simulink model "ReactionWheel"  (R2024a)
settings: Solver=FixedStepAuto  StartTime=0.0  StopTime=60*60  FixedStep=1  RelTol=1e-3
model workspace (MAT data in the model file):
  I_s = [344.15  0  0; 0  344.15  0; 0  0  688.24]
  LocalBodyOffset = [45 0 0]
undefined symbols (not defined in the file): IAU, juliandate, WMM2020
libraries: aerolibutil x16, sharedtransform x6, aerolibtransform2 x4, matrix_library x4, aerolibconvert2 x4, aerolibatmos2 x1, simulink_extras x1, aerolibsatdyn x1, aerolibobsolete x1, aerolibattitudesys x1, simulink x1, vrlib x1
settings Model: Creator=pierc  LastModifiedBy=pierc

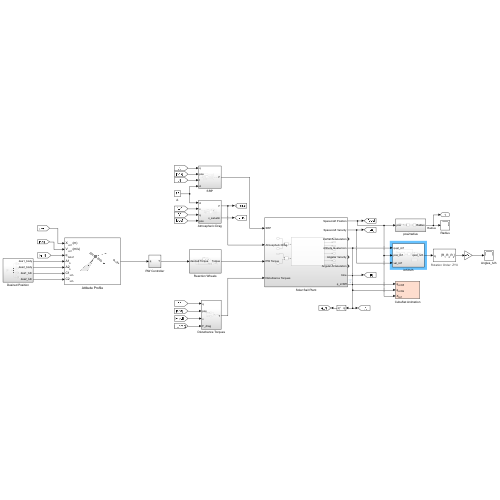
[thumbnail: Simulink's stored preview of the top-level diagram]
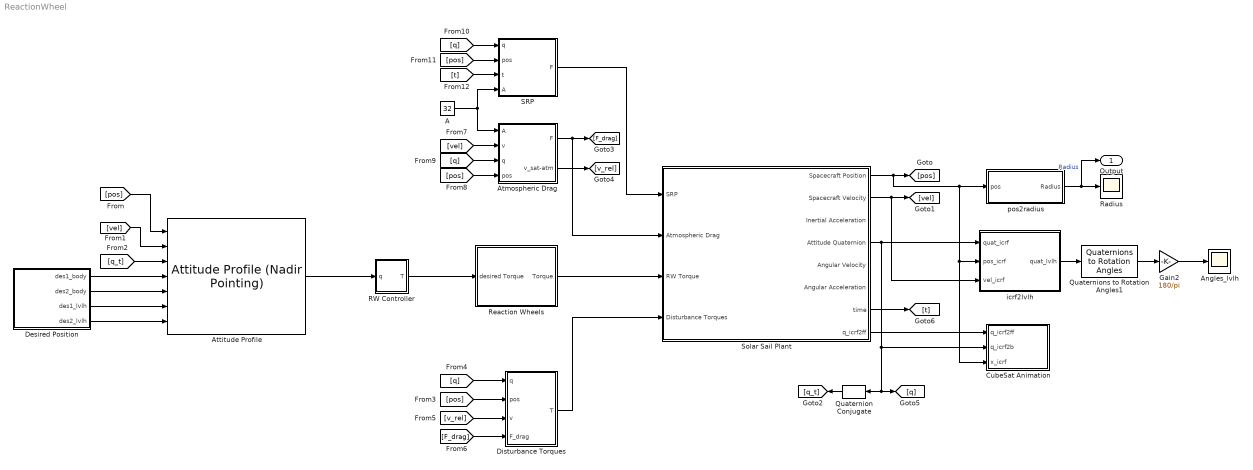
== system ReactionWheel ==
  A : Constant  Value=32
  Angles_lvlh : Scope
  Atmospheric Drag : Subsystem
  "Attitude Profile " : aerolibsatdyn/Attitude Profile (Nadir Pointing)  outputError=on  outputFinalAttitude=off  portFrame=ICRF  pointingMode=Custom  celestialTarget=Sun  tunablePointing=off  primaryAlignmentSrc=Port  primaryAlignment=[0 0 1]  secondaryAlignmentSrc=Port  secondaryAlignment=[1 0 0]  constraintFrame=LVLH  primaryConstraintSrc=Port  primaryConstraint=[1 0 0]  secondaryConstraintSrc=Port  secondaryConstraint=[0 1 0]
  CubeSat Animation : Subsystem  mask(Simulink 3D Animation of CubeSat){enableVis=on, startDate=juliandate(2024, 7, 11, 2, 0, 0), visSampleTime=10, cubesatSize=2e5, showAntenna=on, antennaHeight=1e6, antennaHalfAngle=15}
      mask prompts: enableVis "spacecraft:cubesat:AnimEnableVis"; startDate "spacecraft:cubesat:StartDate"; visSampleTime "spacecraft:cubesat:AnimSampleTime"; cubesatSize "spacecraft:cubesat:MdlSize"; showAntenna "spacecraft:cubesat:ShowCone"; antennaHeight "spacecraft:cubesat:ConeHeight"; antennaHalfAngle "spacecraft:cubesat:ConeAngle"
      mask help: spacecraft:cubesat:VisBlockDesc
      settings: OpenFcn=|
      | if ~builtin('license','test','virtual_reality_toolbox')
      |     set_param(gcb, 'enableVis', 'off');
      | end
      | open_system(gcb,'mask');
      mask Callback enableVis:
      | if strcmp(get_param(gcb,'enableVis'), 'on')
      |     [licAvail, ~] = builtin('license','checkout','Virtual_Reality_Toolbox');
      |     if licAvail
      |         enable = repmat({'on'},7,1);
      |         set_param(gcb, 'Commented', 'off');
      |     else
      |         enable = repmat({'off'},7,1);
      |         set_param(gcb, 'Commented', 'on');
      |         set_param(gcb,'enableVis', 'off');
      |     end
      |     clear licAvail
      | else
      |     enable = repmat({'off'},7,1);
      |     set_param(gcb, 'Commented', 'on');
      | end
      | enable{1} = 'on';
      | set_param(gcb,'MaskEnables', enable);
      | clear enable
      mask Callback showAntenna:
      | if strcmp(get_param(gcb, 'enableVis'), 'on')
      |     enable = get_param(gcb,'MaskEnables');
      |     if strcmp(get_param(gcb, 'showAntenna'), 'off')
      |         enable(6:7) = {'off'};
      |     else
      |         enable(6:7) = {'on'};
      |     end
      |     set_param(gcb,'MaskEnables', enable);
      |     clear enable
      | end
      mask DialogControl enableVis Prompt: Enable visualization with Simulink 3D Animation
      mask DialogControl vrOpenBtn Prompt: spacecraft:cubesat:AnimOpenBtn
      mask DialogControl vrOpenBtn Callback:
      | if builtin('license','checkout','Virtual_Reality_Toolbox')
      |     vrmfunc('FnOpen',getSimulinkBlockHandle([gcb '/VR Sink']));
      | end
      mask DialogControl startDate Prompt: Start date [Julian date]:
      mask DialogControl startDate Tooltip: spacecraft:cubesat:StartDateTT
      mask DialogControl visSampleTime Prompt: Animation refresh rate:
      mask DialogControl visSampleTime Tooltip: spacecraft:cubesat:AnimSampleTimeTT
      mask DialogControl cubesatSize Prompt: CubeSat display size [m]:
      mask DialogControl cubesatSize Tooltip: spacecraft:cubesat:MdlSizeTT
      mask DialogControl Container3 Prompt: spacecraft:cubesat:AntennaPropArea
      mask DialogControl showAntenna Prompt: Show antenna cone in animation
      mask DialogControl showAntenna Tooltip: spacecraft:cubesat:ShowConeTT
      mask DialogControl antennaHeight Prompt: Antenna cone height [m]:
      mask DialogControl antennaHeight Tooltip: spacecraft:cubesat:ConeHeightTT
      mask DialogControl antennaHalfAngle Prompt: Antenna cone half angle [deg]:
      mask DialogControl antennaHalfAngle Tooltip: spacecraft:cubesat:ConeAngleTT
      mask Display:
      | port_label('input', 3, 'X_{icrf}','texmode','on')
      | port_label('input', 2, 'q_{icrf2b}','texmode','on')
      | port_label('input', 1, 'q_{icrf2ff}','texmode','on')
  Desired Position : Subsystem
  Disturbance Torques : Subsystem
  Gain2 : Gain  Gain=180/pi
  Quaternion Conjugate : aerolibutil/Quaternion Conjugate
  Quaternions to Rotation Angles1 : sharedtransform/Quaternions to Rotation Angles  rotationOrder=ZYX  aMode=aMode
  RW Controller : Subsystem
  Radius : Scope
  Reaction Wheels : Subsystem
  SRP : Subsystem
  Solar Sail Plant : Subsystem
  icrf2lvlh : Subsystem
  pos2radius : Subsystem
  Output : Outport
  wires:
  Solar Sail Plant/1(Spacecraft Position) -> icrf2lvlh/2(pos_icrf), CubeSat Animation/3(x_icrf), pos2radius/1(pos), [pos]
  Solar Sail Plant/4(Attitude Quaternion) -> Quaternion Conjugate/1, [q], CubeSat Animation/2(q_icrf2b), icrf2lvlh/1(quat_icrf)
  Solar Sail Plant/8(q_icrf2ff) -> CubeSat Animation/1(q_icrf2ff)
  Gain2/1 -> Angles_lvlh/1
  [pos] -> "Attitude Profile "/1
  Solar Sail Plant/2(Spacecraft Velocity) -> [vel], icrf2lvlh/3(vel_icrf)
  Quaternion Conjugate/1 -> [q_t]
  [q_t] -> "Attitude Profile "/3
  icrf2lvlh/1(quat_lvlh) -> Quaternions to Rotation Angles1/1
  Quaternions to Rotation Angles1/1 -> Gain2/1
  Desired Position/3(des1_lvlh) -> "Attitude Profile "/6
  Desired Position/4(des2_lvlh) -> "Attitude Profile "/7
  "Attitude Profile "/1 -> RW Controller/1(q)
  Desired Position/1(des1_body) -> "Attitude Profile "/4
  Desired Position/2(des2_body) -> "Attitude Profile "/5
  Solar Sail Plant/7(time) -> [t]
  [vel] -> "Attitude Profile "/2
  RW Controller/1(T) -> Reaction Wheels/1(desired Torque)
  Reaction Wheels/1(Torque) -> Solar Sail Plant/3(RW Torque)
  pos2radius/1(Radius) -> Output/1, Radius/1  "Radius"
  [pos] -> Disturbance Torques/2(pos)
  [q] -> Disturbance Torques/1(q)
  [v_rel] -> Disturbance Torques/3(v)
  Disturbance Torques/1(T) -> Solar Sail Plant/4(Disturbance Torques)
  [F_drag] -> Disturbance Torques/4(F_drag)
  [vel] -> Atmospheric Drag/2(v)
  [pos] -> Atmospheric Drag/4(pos)
  [q] -> Atmospheric Drag/3(q)
  Atmospheric Drag/1(F) -> Solar Sail Plant/2(Atmospheric Drag), [F_drag]
  [q] -> SRP/1(q)
  [pos] -> SRP/2(pos)
  [t] -> SRP/3(t)
  A/1 -> Atmospheric Drag/1(A), SRP/4(A)
  Atmospheric Drag/2(v_sat-atm) -> [v_rel]
  SRP/1(F) -> Solar Sail Plant/1(SRP)

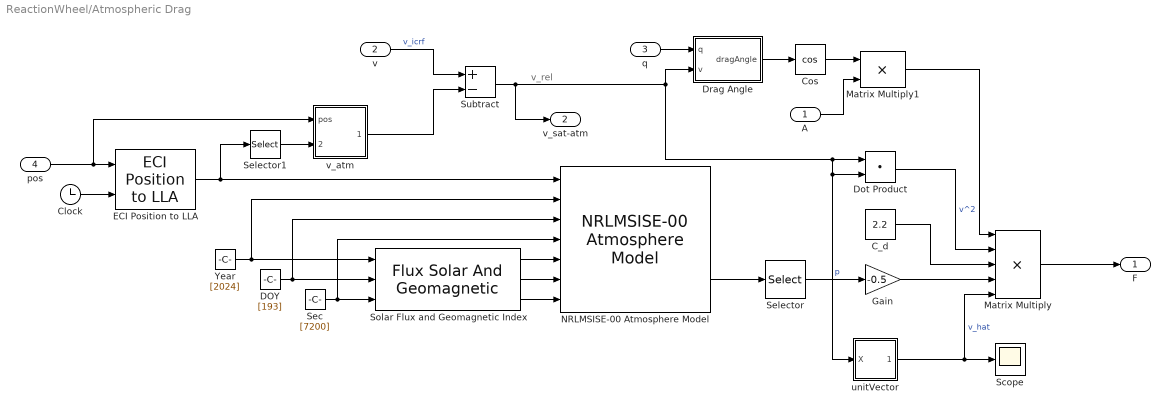
== system ReactionWheel/Atmospheric Drag ==
  note: v_rel
  A : Inport
  v : Inport  Port=2
  q : Inport  Port=3
  pos : Inport  Port=4
  C_d : Constant  Value=2.2
  Clock : Clock
  Cos : Trigonometry  Operator=cos
  DOY : Constant  Value=[193]
  Dot Product : DotProduct  OutDataTypeStr=Inherit: Inherit via internal rule
  Drag Angle : Subsystem
  ECI Position to LLA : aerolibtransform2/ECI Position to LLA  red=IAU-2000/2006  year=2024  month=July  day=11  hour=2  min=0  sec=0  deltaT=Sec  errorflag=Error  extraparamflag=off  eunits=Metric (MKS)  earthmodel=WGS84  flat=1/298.257223563  eqradius=6378137
      settings: AttributesFormatString=%<red>
  Gain : Gain  Gain=-0.5
  Matrix Multiply : Product  Inputs=5
  Matrix Multiply1 : Product
  NRLMSISE-00 Atmosphere Model : aerolibatmos2/NRLMSISE-00 Atmosphere Model  units=Metric (MKS)  lst_input=off  flux_ap_input=on  flags_input=Internal  flags=ones(1,23)  oxygen_in=on  action=Warning
  Scope : Scope
  Sec : Constant  Value=[7200]
  Selector : Selector  InputPortWidth=9  IndexOptions=Index vector (dialog)  Indices=[6]  OutputSizes=1
  Selector1 : Selector  InputPortWidth=3  IndexOptions=Index vector (dialog)  Indices=[1]  OutputSizes=1
  Solar Flux and Geomagnetic Index : FluxSolarAndGeomagnetic
  Subtract : Sum  Inputs=+-
  Year : Constant  Value=[2024]
  unitVector : Subsystem
  v_atm : Subsystem
  F : Outport
  v_sat-atm : Outport  Port=2
  wires:
  NRLMSISE-00 Atmosphere Model/2 -> Selector/1
  ECI Position to LLA/1 -> Selector1/1, NRLMSISE-00 Atmosphere Model/1
  pos/1 -> v_atm/1(pos), ECI Position to LLA/1
  DOY/1 -> NRLMSISE-00 Atmosphere Model/3, Solar Flux and Geomagnetic Index/2
  Solar Flux and Geomagnetic Index/3 -> NRLMSISE-00 Atmosphere Model/7
  Solar Flux and Geomagnetic Index/2 -> NRLMSISE-00 Atmosphere Model/6
  Clock/1 -> ECI Position to LLA/2
  Solar Flux and Geomagnetic Index/1 -> NRLMSISE-00 Atmosphere Model/5
  Gain/1 -> Matrix Multiply/4
  Selector/1 -> Gain/1  "p"
  unitVector/1(X_hat) -> Scope/1, Matrix Multiply/5  "v_hat"
  Cos/1 -> Matrix Multiply1/1
  Drag Angle/1(dragAngle) -> Cos/1
  C_d/1 -> Matrix Multiply/3
  Matrix Multiply1/1 -> Matrix Multiply/1
  q/1 -> Drag Angle/1(q)
  Year/1 -> NRLMSISE-00 Atmosphere Model/2, Solar Flux and Geomagnetic Index/1
  Sec/1 -> NRLMSISE-00 Atmosphere Model/4, Solar Flux and Geomagnetic Index/3
  A/1 -> Matrix Multiply1/2
  Dot Product/1 -> Matrix Multiply/2  "v^2"
  Matrix Multiply/1 -> F/1
  Selector1/1 -> v_atm/2(latitude)
  v_atm/1(v_atm) -> Subtract/2
  Subtract/1 -> Drag Angle/2(v), Dot Product/1, unitVector/1(X), Dot Product/2, v_sat-atm/1
  v/1 -> Subtract/1  "v_icrf"

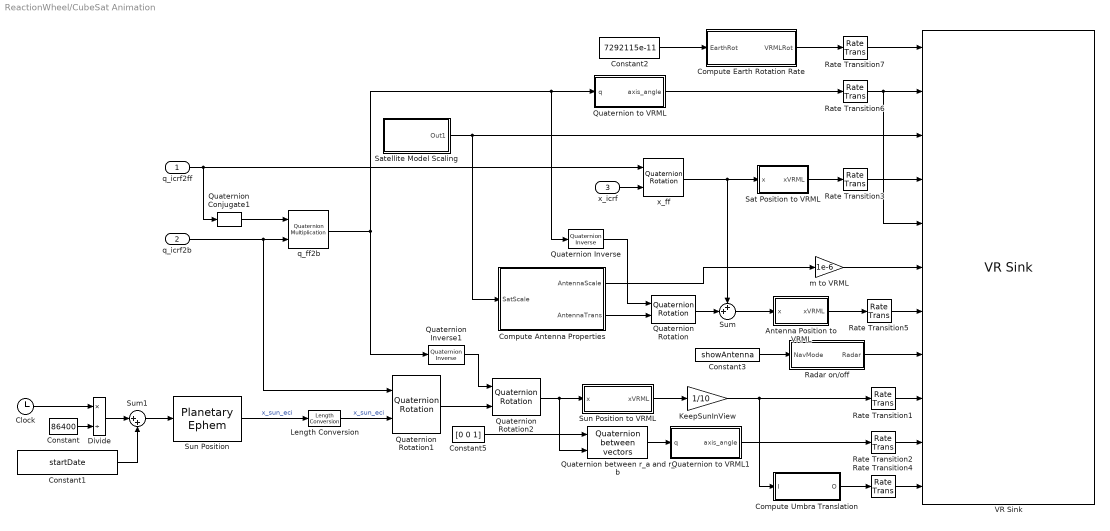
== system ReactionWheel/CubeSat Animation ==
  q_icrf2ff : Inport  PortDimensions=4
  q_icrf2b : Inport  Port=2  PortDimensions=4
  x_icrf : Inport  Port=3  PortDimensions=3
  Antenna Position to VRML : Subsystem
  Clock : Clock
  Compute Antenna Properties : Subsystem
  Compute Earth Rotation Rate : Subsystem
  Compute Umbra Translation : Subsystem
  Constant : Constant  Value=86400
  Constant1 : Constant  Value=startDate  SampleTime=visSampleTime
  Constant2 : Constant  Value=7292115e-11
  Constant3 : Constant  Value=showAntenna
  Constant5 : Constant  Value=[0 0 1]
  Divide : Product  Inputs=*/
  KeepSunInView : Gain  Gain=1/10
  Length Conversion : aerolibconvert2/Length Conversion  IU=km  OU=m
  Quaternion Conjugate1 : aerolibutil/Quaternion Conjugate
  Quaternion Inverse : aerolibutil/Quaternion Inverse
  Quaternion Inverse1 : aerolibutil/Quaternion Inverse
  Quaternion Rotation : aerolibutil/Quaternion Rotation
  Quaternion Rotation1 : aerolibutil/Quaternion Rotation
  Quaternion Rotation2 : aerolibutil/Quaternion Rotation
  Quaternion between r_a and r_b : aerolibattitudesys/Quaternion between vectors
  Quaternion to VRML : Subsystem
  Quaternion to VRML1 : Subsystem
  Radar on/off : Subsystem
  Rate Transition{1..7} (7 alike) : RateTransition
  Sat Position to VRML : Subsystem
  Satellite Model Scaling : Subsystem
  Sum : Sum  Inputs=++|
  Sum1 : Sum  Inputs=|++
  Sun Position : PlanetaryEphem  ephemerisModel=DE421  target=Sun  outputVelocity=off
  Sun Position to VRML : Subsystem
  VR Sink : vrlib/VR Sink  InstantiateOnLoad=on  SampleTime=visSampleTime  ViewEnable=on  RemoteChange=off  RemoteView=off  FieldsWritten=Earth.rotation.4.1.1.double#Satellite.rotation.4.1.1.double#Satellite.scale.3.1.1.double#Satellite.translation.3.1.1.double#AntennaCone.rotation.4.1.1.double#AntennaCone.scale.3.1.1.double#AntennaCone.translation.3.1.1.double#AntennaMaterial.transparency.1.1.1.double#Sun.translation.3.1.1.double#Umbra.rotation.4.1.1.double#Umbra.translation.3.1.1.double  WorldFileName=cubesatAnim.wrl  WorldDescription=CubeSat Orbit Animation  AutoView=off  VideoDimensions=[]  AllowVariableSize=off
  m to VRML : Gain  Gain=1e-6
  q_ff2b : aerolibutil/Quaternion Multiplication
  x_ff : aerolibutil/Quaternion Rotation
  wires:
  Quaternion to VRML1/1(axis_angle) -> Rate Transition2/1
  Quaternion between r_a and r_b/1 -> Quaternion to VRML1/1(q)
  Constant2/1 -> Compute Earth Rotation Rate/1(EarthRot)
  Compute Antenna Properties/1(AntennaScale) -> m to VRML/1
  Quaternion to VRML/1(axis_angle) -> Rate Transition6/1
  Compute Umbra Translation/1(O) -> Rate Transition4/1
  q_icrf2b/1 -> Quaternion Rotation1/1, q_ff2b/2
  Quaternion Rotation2/1 -> Sun Position to VRML/1(x), Quaternion between r_a and r_b/2
  Constant5/1 -> Quaternion between r_a and r_b/1
  KeepSunInView/1 -> Compute Umbra Translation/1(I), Rate Transition1/1
  Sun Position to VRML/1(xVRML) -> KeepSunInView/1
  Sat Position to VRML/1(xVRML) -> Rate Transition3/1
  Compute Antenna Properties/2(AntennaTrans) -> Quaternion Rotation/2
  Satellite Model Scaling/1(Out1) -> VR Sink/3, Compute Antenna Properties/1(SatScale)
  Constant3/1 -> Radar on/off/1(NavMode)
  q_ff2b/1 -> Quaternion Inverse/1, Quaternion to VRML/1(q), Quaternion Inverse1/1
  Quaternion Rotation1/1 -> Quaternion Rotation2/2
  Compute Earth Rotation Rate/1(VRMLRot) -> Rate Transition7/1
  Antenna Position to VRML/1(xVRML) -> Rate Transition5/1
  Quaternion Inverse/1 -> Quaternion Rotation/1
  x_ff/1 -> Sum/1, Sat Position to VRML/1(x)
  Quaternion Rotation/1 -> Sum/2
  Sum/1 -> Antenna Position to VRML/1(x)
  Quaternion Inverse1/1 -> Quaternion Rotation2/1
  Rate Transition4/1 -> VR Sink/11
  Rate Transition2/1 -> VR Sink/10
  Rate Transition1/1 -> VR Sink/9
  Rate Transition5/1 -> VR Sink/7
  m to VRML/1 -> VR Sink/6
  Rate Transition3/1 -> VR Sink/4
  Rate Transition7/1 -> VR Sink/1
  Rate Transition6/1 -> VR Sink/5, VR Sink/2
  Constant1/1 -> Sum1/2
  Divide/1 -> Sum1/1
  Constant/1 -> Divide/2
  Sun Position/1 -> Length Conversion/1  "x_sun_eci"
  Clock/1 -> Divide/1
  Length Conversion/1 -> Quaternion Rotation1/2  "x_sun_eci"
  Sum1/1 -> Sun Position/1
  Radar on/off/1(Radar) -> VR Sink/8
  Quaternion Conjugate1/1 -> q_ff2b/1
  q_icrf2ff/1 -> Quaternion Conjugate1/1, x_ff/1
  x_icrf/1 -> x_ff/2

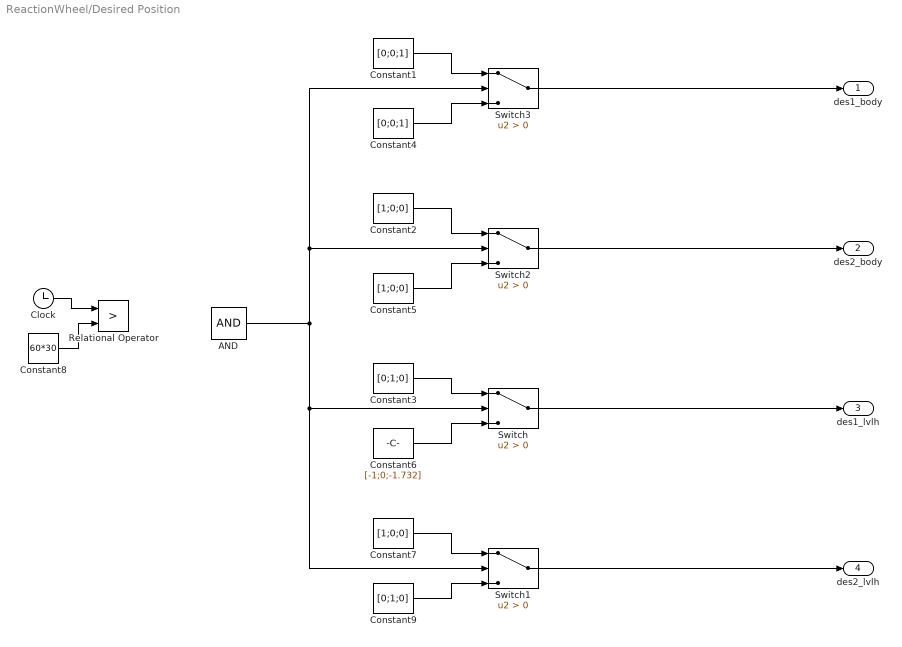
== system ReactionWheel/Desired Position ==
  AND : Logic  IconShape=distinctive  AllPortsSameDT=off  OutDataTypeStr=boolean
  Clock : Clock
  Constant1 : Constant  Value=[0;0;1]
  Constant2 : Constant  Value=[1;0;0]
  Constant3 : Constant  Value=[0;1;0]
  Constant4 : Constant  Value=[0;0;1]
  Constant5 : Constant  Value=[1;0;0]
  Constant6 : Constant  Value=[-1;0;-1.732]
  Constant7 : Constant  Value=[1;0;0]
  Constant8 : Constant  Value=60*30
  Constant9 : Constant  Value=[0;1;0]
  Relational Operator : RelationalOperator  Operator=>  OutDataTypeStr=boolean  RndMeth=Simplest  InputSameDT=off
  Switch{,1..3} (4 alike) : Switch  Criteria=u2 > Threshold  SaturateOnIntegerOverflow=off  InputSameDT=off
  des1_body : Outport
  des2_body : Outport  Port=2
  des1_lvlh : Outport  Port=3
  des2_lvlh : Outport  Port=4
  wires:
  Constant8/1 -> Relational Operator/2
  Constant6/1 -> Switch/3
  Clock/1 -> Relational Operator/1
  Constant9/1 -> Switch1/3
  Constant4/1 -> Switch3/3
  Constant5/1 -> Switch2/3
  Switch3/1 -> des1_body/1
  Switch2/1 -> des2_body/1
  Switch/1 -> des1_lvlh/1
  Switch1/1 -> des2_lvlh/1
  Constant1/1 -> Switch3/1
  Constant2/1 -> Switch2/1
  Constant7/1 -> Switch1/1
  Constant3/1 -> Switch/1
  AND/1 -> Switch/2, Switch1/2, Switch3/2, Switch2/2

== system ReactionWheel/Disturbance Torques ==
  q : Inport
  pos : Inport  Port=2
  v : Inport  Port=3
  F_drag : Inport  Port=4
  Add : Sum
  Atmospheric Drag Torque : Subsystem
  Magnetic Field Torque : Subsystem
  T : Outport
  wires:
  pos/1 -> Magnetic Field Torque/1(pos)
  v/1 -> Atmospheric Drag Torque/1(v)
  q/1 -> Atmospheric Drag Torque/2(q), Magnetic Field Torque/2(q)
  Atmospheric Drag Torque/1(T) -> Add/1
  Magnetic Field Torque/1(T) -> Add/2
  Add/1 -> T/1  "T"
  F_drag/1 -> Atmospheric Drag Torque/3(F_drag)

== system ReactionWheel/RW Controller ==
  q : Inport
  Constant : Constant  Value=-0.001
  Constant1 : Constant  Value=0.001
  Demo Controller : slpidlib/PID Controller  Controller=PD  Form=Parallel  TimeDomain=Discrete-time  UseExternalTs=off  SampleTime=-1  IntegratorMethod=Trapezoidal  FilterMethod=Trapezoidal  ControllerParametersSource=internal  P=.0001  I=0  UseKiTs=off  D=.017  UseExternalDerivativeSource=off  N=1  UseFilter=off  TunerSelectOption=Transfer Function Based (PID Tuner App)  InitialConditionSource=internal  InitialConditionForIntegrator=0  InitialConditionForFilter=0  DifferentiatorICPrevScaledInput=0  ExternalReset=none  TrackingMode=off  Kt=1  LimitOutput=on  SatLimitsSource=internal  UpperSaturationLimit=0.008  LowerSaturationLimit=-0.008  LinearizeAsGain=on  AntiWindupMode=none  Kb=1  LimitIntegrator=off  UpperIntegratorSaturationLimit=inf  LowerIntegratorSaturationLimit=-inf  POutMin=[]  POutMax=[]  IOutMin=[]  IOutMax=[]  DOutMin=[]  DOutMax=[]  NOutMin=[]  NOutMax=[]  SumOutMin=[]  SumOutMax=[]  SaturationOutMin=[]  SaturationOutMax=[]  PParamMin=[]  PParamMax=[]  IParamMin=[]  IParamMax=[]  DParamMin=[]  DParamMax=[]  NParamMin=[]  NParamMax=[]  KbParamMin=[]  KbParamMax=[]  KtParamMin=[]  KtParamMax=[]  KbOutMin=[]  KbOutMax=[]  KtOutMin=[]  KtOutMax=[]  IntegratorOutMin=[]  IntegratorOutMax=[]  FilterOutMin=[]  FilterOutMax=[]  SumI1OutMin=[]  SumI1OutMax=[]  SumI2OutMin=[]  SumI2OutMax=[]  SumI3OutMin=[]  SumI3OutMax=[]  SumI4OutMin=[]  SumI4OutMax=[]  SumDOutMin=[]  SumDOutMax=[]  DifferentiatorOutMin=[]  DifferentiatorOutMax=[]  FilterDiffOutCoefMin=[]  FilterDiffOutCoefMax=[]  ReciprocalOutMin=[]  ReciprocalOutMax=[]  SumDenOutMin=[]  SumDenOutMax=[]  SumNumOutMin=[]  SumNumOutMax=[]  DivideOutMin=[]  DivideOutMax=[]  UdiffTsProdOutMin=[]  UdiffTsProdOutMax=[]  NTsProdOutMin=[]  NTsProdOutMax=[]  UintegralTsProdOutMin=[]  UintegralTsProdOutMax=[]  UngainTsProdOutMin=[]  UngainTsProdOutMax=[]  ClampingZeroOutDataTypeStr=Inherit: Inherit via back propagation  ClampingZeroOutMin=[]  ClampingZeroOutMax=[]  FilterDenConstantOutDataTypeStr=Inherit: Inherit via back propagation  FilterDenConstantOutMin=[]  FilterDenConstantOutMax=[]  PCopyOutDataTypeStr=Inherit: Inherit via back propagation  PCopyOutMin=[]  PCopyOutMax=[]  NCopyOutDataTypeStr=Inherit: Inherit via back propagation  NCopyOutMin=[]  NCopyOutMax=[]  IntegratorContinuousStateAttributes=''  IntegratorStateMustResolveToSignalObject=off  IntegratorRTWStateStorageClass=Auto  FilterContinuousStateAttributes=''  FilterStateMustResolveToSignalObject=off  FilterRTWStateStorageClass=Auto  ParallelPVariant=InternalParameters  IdealPVariant=Disabled  IVariant=Disabled  DVariant=InternalParameters  IntegratorVariant=Disabled  SatVariant=Enabled  AWVariant=Disabled  PCopyVariant=Disabled  TRVariant=Disabled  FdbkBlocksVariant=Forward  IdealPFdbkVariant=Disabled  SatFdbkVariant=Disabled  DerivativeFilterVariant=Differentiator  NVariant=Passthrough  NCopyVariant=Disabled_SignalSpec  FilterICVariant=InternalICsDifferentiator  IntegratorICVariant=Disabled  ExternalResetVariant=Disabled  TRSumVariant=Passthrough  SumFdbkVariant=Disabled  SumVariant=Sum_PD  TsampFilterVariant=InternalTs  TsampNgainVariant=Passthrough  TsampIntegralVariant=Disabled_SignalSpec  ExternalSaturationOutDataTypeStr=Inherit: Same as second input  DerivativeSourceVariant=ErrorSignal
  Max : MinMax  Function=max  Inputs=2
  Min : MinMax  Inputs=2
  Quaternions to Rotation Angles : sharedtransform/Quaternions to Rotation Angles  rotationOrder=XYZ  aMode=aMode
  T : Outport
  wires:
  q/1 -> Quaternions to Rotation Angles/1
  Quaternions to Rotation Angles/1 -> Demo Controller/1
  Constant/1 -> Max/1
  Demo Controller/1 -> Max/2
  Constant1/1 -> Min/1
  Max/1 -> Min/2
  Min/1 -> T/1

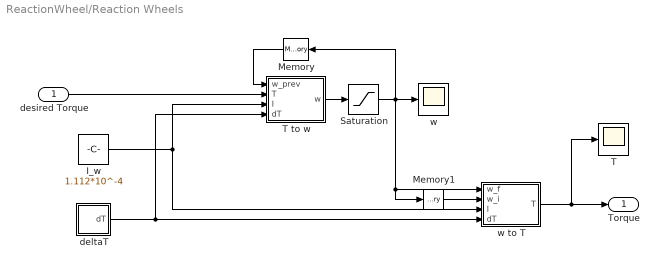
== system ReactionWheel/Reaction Wheels ==
  desired Torque : Inport
  I_w : Constant  Value=1.112*10^-4
  Memory : Memory
  Memory1 : Memory
  Saturation : Saturate  UpperLimit=1017  LowerLimit=-1017
  T : Scope
  T to w : Subsystem
  deltaT : Subsystem
  w : Scope
  w to T : Subsystem
  Torque : Outport
  wires:
  Saturation/1 -> w/1, Memory1/1, w to T/1(w_f), Memory/1
  Memory1/1 -> w to T/2(w_i)
  I_w/1 -> w to T/3(I), T to w/3(I)
  T to w/1(w) -> Saturation/1
  deltaT/1(dT) -> T to w/4(dT), w to T/4(dT)
  desired Torque/1 -> T to w/2(T)
  Memory/1 -> T to w/1(w_prev)
  w to T/1(T) -> Torque/1, T/1

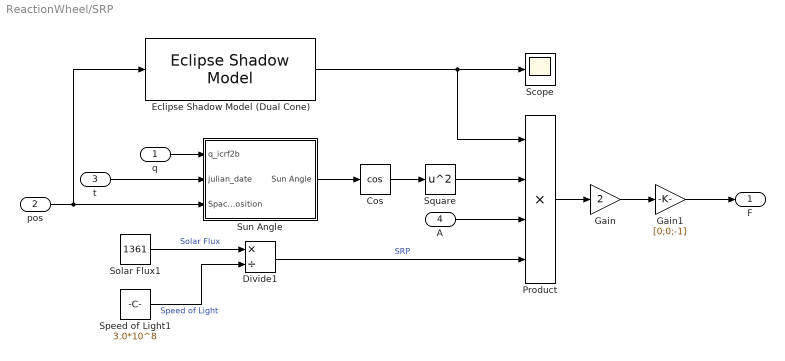
== system ReactionWheel/SRP ==
  q : Inport
  pos : Inport  Port=2
  t : Inport  Port=3
  A : Inport  Port=4
  Cos : Trigonometry  Operator=cos
  Divide1 : Product  Inputs=*/
  Eclipse Shadow Model (Dual Cone) : EclipseShadowModel  startDate=juliandate(2024, 7, 11,2,0,0)  ephemerisModel=DE432t  ephemerisStartDate=juliandate(2024, 7, 11,2,0,0)  ephemerisEndDate=juliandate(2024, 7, 12,2,0,0)
  Gain : Gain  Gain=2
  Gain1 : Gain  Gain=[0;0;-1]
  Product : Product  Inputs=4
  Scope : Scope
  Solar Flux1 : Constant  Value=1361
  Speed of Light1 : Constant  Value=3.0*10^8
  Square : Math  Operator=square
  Sun Angle : Subsystem
  F : Outport
  wires:
  pos/1 -> Eclipse Shadow Model (Dual Cone)/1, Sun Angle/3(Spacecraft Position)
  q/1 -> Sun Angle/1(q_icrf2b)
  t/1 -> Sun Angle/2(julian_date)
  Solar Flux1/1 -> Divide1/1  "Solar Flux"
  Speed of Light1/1 -> Divide1/2  "Speed of Light"
  Sun Angle/1(Sun Angle) -> Cos/1
  Cos/1 -> Square/1
  Square/1 -> Product/2
  A/1 -> Product/3
  Divide1/1 -> Product/4  "SRP"
  Product/1 -> Gain/1
  Gain/1 -> Gain1/1
  Gain1/1 -> F/1
  Eclipse Shadow Model (Dual Cone)/1 -> Scope/1, Product/1

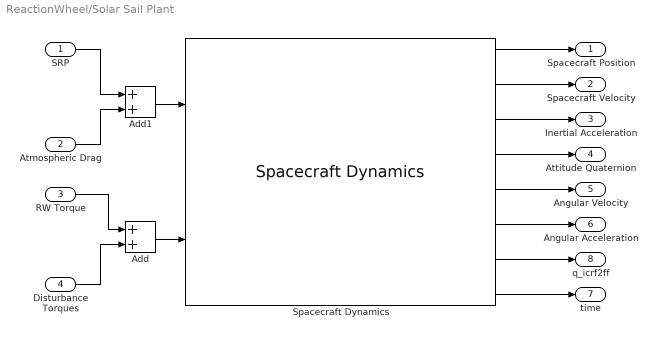
== system ReactionWheel/Solar Sail Plant ==
  SRP : Inport
  Atmospheric Drag : Inport  Port=2
  RW Torque : Inport  Port=3
  Disturbance Torques : Inport  Port=4
  Add : Sum
  Add1 : Sum
  Spacecraft Dynamics : SpacecraftDynamics  outputAccel=on  startDate=juliandate(2024, 7, 11, 2, 0, 0)  mass=4.93  inertia=[3.79,-1.90*10^-4,-8.18*10^-4;-1.90*10^-4,3.79,1.47*10^-3;-8.18*10^-4,1.47*10^-3,7.33]  semiMajorAxis=7078140  eccentricity=0.001  inclination=98.1928  raan=22  argPeriapsis=360  trueAnomaly=0  attitude=[0.7,-0.1915,-0.6337,-0.2677]  outputAngAccel=on  outputTransform=on  ephemerisModel=DE432t  ephemerisStartDate=juliandate(2024, 7, 11, 2, 0, 0)  ephemerisEndDate=juliandate(2025, 1, 1, 0, 0, 0)  useThirdBodyGravity=on  useSRP=on  srpArea=32
  Spacecraft Position : Outport
  Spacecraft Velocity : Outport  Port=2
  Inertial Acceleration : Outport  Port=3
  Attitude Quaternion : Outport  Port=4
  Angular Velocity : Outport  Port=5
  Angular Acceleration : Outport  Port=6
  time : Outport  Port=7
  q_icrf2ff : Outport  Port=8
  wires:
  Spacecraft Dynamics/1 -> Spacecraft Position/1
  Spacecraft Dynamics/2 -> Spacecraft Velocity/1
  Spacecraft Dynamics/3 -> Inertial Acceleration/1
  Spacecraft Dynamics/4 -> Attitude Quaternion/1
  Spacecraft Dynamics/5 -> Angular Velocity/1
  Spacecraft Dynamics/6 -> Angular Acceleration/1
  Spacecraft Dynamics/8 -> time/1
  Spacecraft Dynamics/7 -> q_icrf2ff/1
  RW Torque/1 -> Add/1
  Add/1 -> Spacecraft Dynamics/2
  Disturbance Torques/1 -> Add/2
  Add1/1 -> Spacecraft Dynamics/1
  SRP/1 -> Add1/1
  Atmospheric Drag/1 -> Add1/2

== system ReactionWheel/icrf2lvlh ==
  quat_icrf : Inport
  pos_icrf : Inport  Port=2
  vel_icrf : Inport  Port=3
  DCM_icrf2lvlh : Subsystem
  Direction Cosine Matrix to Quaternions : sharedtransform/Direction Cosine Matrix  to Quaternions  aMode=0  action=Warning  tolerance=eps(4)
      settings: LibrarySourceBlock=|
      | aerolibtransform2/Direction Cosine Matrix
      | to Quaternions
  MATLAB Function : MATLAB Function  Commented=on  TreatAsAtomicUnit=on
  Quaternion Multiplication : aerolibutil/Quaternion Multiplication
  quat_lvlh : Outport
  wires:
  quat_icrf/1 -> Quaternion Multiplication/2
  Direction Cosine Matrix to Quaternions/1 -> Quaternion Multiplication/1
  Quaternion Multiplication/1 -> quat_lvlh/1
  DCM_icrf2lvlh/1(DCM) -> Direction Cosine Matrix to Quaternions/1
  pos_icrf/1 -> DCM_icrf2lvlh/1(pos)
  vel_icrf/1 -> DCM_icrf2lvlh/2(vel)

== system ReactionWheel/pos2radius ==
  pos : Inport
  Dot Product : DotProduct  OutDataTypeStr=Inherit: Inherit via internal rule
  Square Root : Sqrt
  Radius : Outport
  wires:
  pos/1 -> Dot Product/2, Dot Product/1
  Dot Product/1 -> Square Root/1
  Square Root/1 -> Radius/1  "Radius"

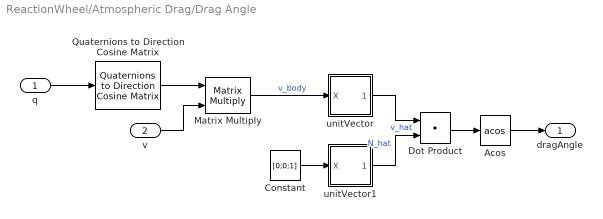
== system ReactionWheel/Atmospheric Drag/Drag Angle ==
  q : Inport
  v : Inport  Port=2
  Acos : Trigonometry  Operator=acos
  Constant : Constant  Value=[0;0;1]
  Dot Product : DotProduct  OutDataTypeStr=Inherit: Inherit via internal rule
  Matrix Multiply : Product  Multiplication=Matrix(*)
  Quaternions to Direction Cosine Matrix : sharedtransform/Quaternions to  Direction Cosine Matrix  aMode=aMode
      settings: LibrarySourceBlock=|
      | aerolibtransform2/Quaternions to
      | Direction Cosine Matrix
  unitVector : Subsystem
  unitVector1 : Subsystem
  dragAngle : Outport
  wires:
  q/1 -> Quaternions to Direction Cosine Matrix/1
  Quaternions to Direction Cosine Matrix/1 -> Matrix Multiply/1
  v/1 -> Matrix Multiply/2
  Matrix Multiply/1 -> unitVector/1(X)  "v_body"
  Constant/1 -> unitVector1/1(X)
  unitVector/1(X_hat) -> Dot Product/1  "v_hat"
  unitVector1/1(X_hat) -> Dot Product/2  "N_hat"
  Dot Product/1 -> Acos/1
  Acos/1 -> dragAngle/1

== system ReactionWheel/Atmospheric Drag/unitVector ==
  X : Inport
  Divide : Product  Inputs=*/
  Dot Product : DotProduct  OutDataTypeStr=Inherit: Inherit via internal rule
  Square Root : Sqrt
  X_hat : Outport
  wires:
  X/1 -> Divide/1, Dot Product/2, Dot Product/1
  Dot Product/1 -> Square Root/1
  Square Root/1 -> Divide/2
  Divide/1 -> X_hat/1

== system ReactionWheel/Atmospheric Drag/v_atm ==
  pos : Inport
  latitude : Inport  Port=2
  Cos : Trigonometry  Operator=cos
  Cross Product : matrix_library/Cross Product
  Degrees to Radians : simulink_extras/Transformations/Degrees to Radians
  Divide : Product  Inputs=**
  Earth Angular Vel : Constant  Value=2*pi/86400
  Multiply1 : Gain  Gain=[0;0;1]
  v_atm : Outport
  wires:
  pos/1 -> Cross Product/2
  latitude/1 -> Degrees to Radians/1
  Cos/1 -> Divide/2
  Divide/1 -> Multiply1/1
  Multiply1/1 -> Cross Product/1  "rotational velocity"
  Cross Product/1 -> v_atm/1
  Degrees to Radians/1 -> Cos/1
  Earth Angular Vel/1 -> Divide/1

== system ReactionWheel/CubeSat Animation/Antenna Position to VRML ==
  x : Inport
  ECEF to VRML : Subsystem
  Length Conversion : aerolibconvert2/Length Conversion  IU=m  OU=km
  km to VRML units : Gain  Gain=1/1000
  xVRML : Outport  VectorParamsAs1DForOutWhenUnconnected=off
  wires:
  Length Conversion/1 -> km to VRML units/1
  km to VRML units/1 -> ECEF to VRML/1(M)
  x/1 -> Length Conversion/1
  ECEF to VRML/1(VR) -> xVRML/1

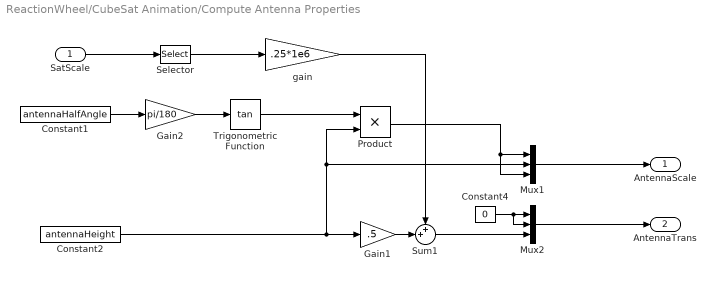
== system ReactionWheel/CubeSat Animation/Compute Antenna Properties ==
  SatScale : Inport
  Constant1 : Constant  Value=antennaHalfAngle
  Constant2 : Constant  Value=antennaHeight
  Constant4 : Constant  Value=0
  Gain1 : Gain  Gain=.5
  Gain2 : Gain  Gain=pi/180
  Mux1 : Mux  Inputs=3
  Mux2 : Mux  Inputs=3
  Product : Product
  Selector : Selector  InputPortWidth=3  IndexOptions=Index vector (dialog)  Indices=1  OutputSizes=1
  Sum1 : Sum  Inputs=++|
  Trigonometric Function : Trigonometry  Operator=tan
  gain : Gain  Gain=.25*1e6
  AntennaScale : Outport  VectorParamsAs1DForOutWhenUnconnected=off
  AntennaTrans : Outport  Port=2  VectorParamsAs1DForOutWhenUnconnected=off
  wires:
  Gain2/1 -> Trigonometric Function/1
  Constant4/1 -> Mux2/1, Mux2/2
  Sum1/1 -> Mux2/3
  Constant2/1 -> Gain1/1, Mux1/2, Product/2
  gain/1 -> Sum1/1
  Constant1/1 -> Gain2/1
  Product/1 -> Mux1/3, Mux1/1
  Gain1/1 -> Sum1/2
  Trigonometric Function/1 -> Product/1
  Mux2/1 -> AntennaTrans/1
  Mux1/1 -> AntennaScale/1
  SatScale/1 -> Selector/1
  Selector/1 -> gain/1

== system ReactionWheel/CubeSat Animation/Compute Earth Rotation Rate ==
  EarthRot : Inport
  Constant : Constant  Value=0
  Constant1 : Constant  Value=0
  Euler Angles to Quaternions : aerolibobsolete/Euler Angles to Quaternions
  Quaternion to VRML : Subsystem
  Sum : Sum  Inputs=|++
  Unit Delay : UnitDelay  SampleTime=-1  HasFrameUpgradeWarning=on
  Vector Concatenate : Concatenate  NumInputs=3
  VRMLRot : Outport  VectorParamsAs1DForOutWhenUnconnected=off
  wires:
  Quaternion to VRML/1(AxisAngle) -> VRMLRot/1
  Euler Angles to Quaternions/1 -> Quaternion to VRML/1(q)
  Vector Concatenate/1 -> Euler Angles to Quaternions/1
  Constant1/1 -> Vector Concatenate/2
  Constant/1 -> Vector Concatenate/1
  Sum/1 -> Unit Delay/1, Vector Concatenate/3
  Unit Delay/1 -> Sum/2
  EarthRot/1 -> Sum/1

== system ReactionWheel/CubeSat Animation/Compute Umbra Translation ==
  I : Inport
  Add : Sum
  ConeHalfLength : Gain  Gain=692
  InvertSunPosECEF : Gain  Gain=-1
  unitVec : Subsystem
  O : Outport  VectorParamsAs1DForOutWhenUnconnected=off
  wires:
  ConeHalfLength/1 -> Add/2
  I/1 -> InvertSunPosECEF/1
  Add/1 -> O/1
  InvertSunPosECEF/1 -> unitVec/1(I), Add/1
  unitVec/1(O) -> ConeHalfLength/1

== system ReactionWheel/CubeSat Animation/Quaternion to VRML ==
  q : Inport
  Demux : Demux
  "Flip 180 deg, rotate 90" : Constant  Value=[0 -.7071 .7071 0]
  Gain : Gain  Gain=2
  Mux : Mux
  Quaternion Multiplication : aerolibutil/Quaternion Multiplication
  Selector : Selector  InputPortWidth=4  IndexOptions=Index vector (dialog)  Indices=[3 4 2 1]  OutputSizes=1
  Trigonometric Function : Trigonometry  Operator=acos
  axis_angle : Outport  VectorParamsAs1DForOutWhenUnconnected=off
  wires:
  Demux/4 -> Mux/4
  Demux/3 -> Mux/3
  Demux/2 -> Mux/2
  Gain/1 -> Mux/1
  Selector/1 -> axis_angle/1
  q/1 -> Quaternion Multiplication/1
  Mux/1 -> Selector/1
  Trigonometric Function/1 -> Gain/1
  Demux/1 -> Trigonometric Function/1
  "Flip 180 deg, rotate 90"/1 -> Quaternion Multiplication/2
  Quaternion Multiplication/1 -> Demux/1

== system ReactionWheel/CubeSat Animation/Quaternion to VRML1 ==
  q : Inport
  Demux : Demux
  "Flip 180 deg, rotate 90" : Constant  Value=[0 -0.7071 0.7071 0]
  Gain : Gain  Gain=2
  Mux : Mux
  Quaternion Multiplication : aerolibutil/Quaternion Multiplication
  Selector : Selector  InputPortWidth=4  IndexOptions=Index vector (dialog)  Indices=[3 4 2 1]  OutputSizes=1
  Trigonometric Function : Trigonometry  Operator=acos
  axis_angle : Outport  VectorParamsAs1DForOutWhenUnconnected=off
  wires:
  Demux/4 -> Mux/4
  Demux/3 -> Mux/3
  Demux/2 -> Mux/2
  Gain/1 -> Mux/1
  Selector/1 -> axis_angle/1
  Mux/1 -> Selector/1
  Trigonometric Function/1 -> Gain/1
  Demux/1 -> Trigonometric Function/1
  "Flip 180 deg, rotate 90"/1 -> Quaternion Multiplication/2
  q/1 -> Quaternion Multiplication/1
  Quaternion Multiplication/1 -> Demux/1

== system ReactionWheel/CubeSat Animation/Radar on//off ==
  NavMode : Inport
  Add : Sum  Inputs=-+
  Compare To Constant : simulink/Logic and Bit Operations/Compare To Constant  relop===  const=1  OutDataTypeStr=boolean  ZeroCross=off
  Constant : Constant
  Data Type Conversion : DataTypeConversion  OutDataTypeStr=double  SaturateOnIntegerOverflow=off  RndMeth=Floor
  Gain : Gain  Gain=0.6
  Radar : Outport  VectorParamsAs1DForOutWhenUnconnected=off
  wires:
  NavMode/1 -> Compare To Constant/1
  Compare To Constant/1 -> Data Type Conversion/1
  Data Type Conversion/1 -> Gain/1
  Gain/1 -> Add/1
  Constant/1 -> Add/2
  Add/1 -> Radar/1

== system ReactionWheel/CubeSat Animation/Sat Position to VRML ==
  x : Inport
  ECEF to VRML : Subsystem
  Length Conversion : aerolibconvert2/Length Conversion  IU=m  OU=km
  km to VRML units : Gain  Gain=1/1000
  xVRML : Outport  VectorParamsAs1DForOutWhenUnconnected=off
  wires:
  ECEF to VRML/1(VR) -> xVRML/1
  x/1 -> Length Conversion/1
  km to VRML units/1 -> ECEF to VRML/1(M)
  Length Conversion/1 -> km to VRML units/1

== system ReactionWheel/CubeSat Animation/Satellite Model Scaling ==
  Constant : Constant  Value=cubesatSize
  Mux : Mux  Inputs=3
  ScaleModelToVRML : Gain  Gain=1/.3e6
  Out1 : Outport  VectorParamsAs1DForOutWhenUnconnected=off
  wires:
  ScaleModelToVRML/1 -> Mux/3, Mux/1, Mux/2
  Constant/1 -> ScaleModelToVRML/1
  Mux/1 -> Out1/1

== system ReactionWheel/CubeSat Animation/Sun Position to VRML ==
  x : Inport
  ECEF to VRML : Subsystem
  Length Conversion : aerolibconvert2/Length Conversion  IU=m  OU=km
  km to VRML units : Gain  Gain=1/1000
  xVRML : Outport  VectorParamsAs1DForOutWhenUnconnected=off
  wires:
  ECEF to VRML/1(VR) -> xVRML/1
  x/1 -> Length Conversion/1
  km to VRML units/1 -> ECEF to VRML/1(M)
  Length Conversion/1 -> km to VRML units/1

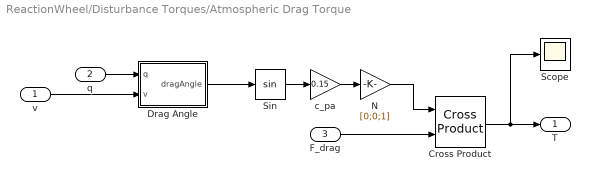
== system ReactionWheel/Disturbance Torques/Atmospheric Drag Torque ==
  v : Inport
  q : Inport  Port=2
  F_drag : Inport  Port=3
  Cross Product : matrix_library/Cross Product
  Drag Angle : Subsystem
  N : Gain  Gain=[0;0;1]
  Scope : Scope
  Sin : Trigonometry
  c_pa : Gain  Gain=0.15
  T : Outport
  wires:
  v/1 -> Drag Angle/2(v)
  q/1 -> Drag Angle/1(q)
  Drag Angle/1(dragAngle) -> Sin/1
  Sin/1 -> c_pa/1
  c_pa/1 -> N/1
  Cross Product/1 -> T/1, Scope/1
  N/1 -> Cross Product/1
  F_drag/1 -> Cross Product/2

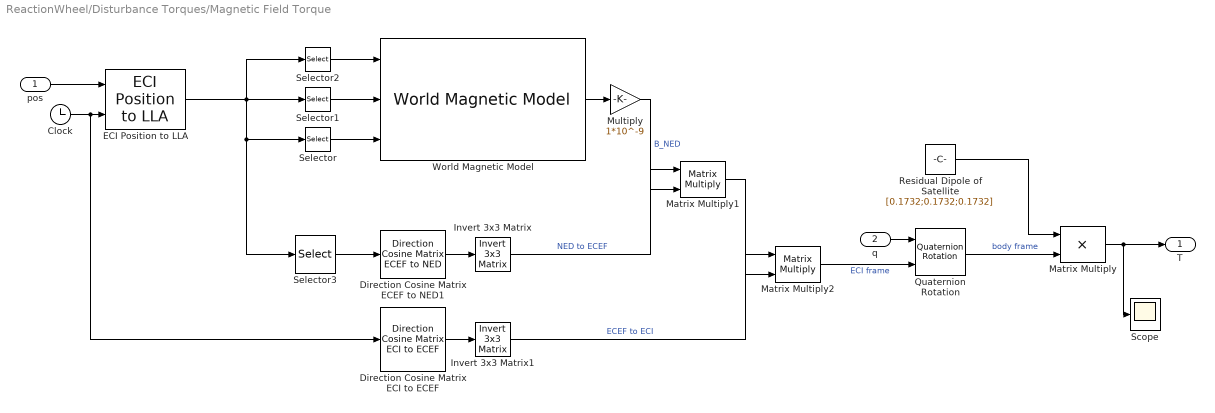
== system ReactionWheel/Disturbance Torques/Magnetic Field Torque ==
  pos : Inport
  q : Inport  Port=2
  Clock : Clock
  Direction Cosine Matrix ECEF to NED1 : aerolibtransform2/Direction Cosine Matrix ECEF to NED
  Direction Cosine Matrix ECI to ECEF : aerolibtransform2/Direction Cosine Matrix ECI to ECEF  red=IAU-2000/2006  year=2024  month=July  day=11  hour=2  min=0  sec=0  deltaT=Sec  errorflag=Error  extraparamflag=off
      settings: AttributesFormatString=%<red>
  ECI Position to LLA : aerolibtransform2/ECI Position to LLA  red=IAU-2000/2006  year=2024  month=July  day=11  hour=2  min=0  sec=0  deltaT=Sec  errorflag=Error  extraparamflag=off  eunits=Metric (MKS)  earthmodel=WGS84  flat=1/298.257223563  eqradius=6378137
      settings: AttributesFormatString=%<red>
  Invert 3x3 Matrix : aerolibutil/Invert  3x3 Matrix
  Invert 3x3 Matrix1 : aerolibutil/Invert  3x3 Matrix
  Matrix Multiply : Product
  Matrix Multiply1 : Product  Multiplication=Matrix(*)
  Matrix Multiply2 : Product  Multiplication=Matrix(*)
  Multiply : Gain  Gain=1*10^-9
  Quaternion Rotation : aerolibutil/Quaternion Rotation
  Residual Dipole of Satellite : Constant  Value=[0.1732;0.1732;0.1732]
  Scope : Scope
  Selector : Selector  InputPortWidth=3  IndexOptions=Index vector (dialog)  Indices=[2]  OutputSizes=1
  Selector1 : Selector  InputPortWidth=3  IndexOptions=Index vector (dialog)  Indices=[1]  OutputSizes=1
  Selector2 : Selector  InputPortWidth=3  IndexOptions=Index vector (dialog)  Indices=[3]  OutputSizes=1
  Selector3 : Selector  InputPortWidth=3  IndexOptions=Index vector (dialog)  Indices=[1 2]  OutputSizes=1
  World Magnetic Model : aerolibgravity2/World Magnetic Model  model=WMM2020 (2020-2025)  customFile='WMM2020.COF'  units=Metric (MKS)  time_in=off  month=July  day=11  year=2024  action=Error  h_out=off  dec_out=off  inc_out=off  ti_out=off
  T : Outport
  wires:
  Clock/1 -> Direction Cosine Matrix ECI to ECEF/1, ECI Position to LLA/2
  pos/1 -> ECI Position to LLA/1
  Selector/1 -> World Magnetic Model/3
  Selector1/1 -> World Magnetic Model/2
  ECI Position to LLA/1 -> Selector3/1, Selector/1, Selector2/1, Selector1/1
  Selector2/1 -> World Magnetic Model/1
  World Magnetic Model/1 -> Multiply/1
  Residual Dipole of Satellite/1 -> Matrix Multiply/1
  Matrix Multiply/1 -> Scope/1, T/1
  Selector3/1 -> Direction Cosine Matrix ECEF to NED1/1
  Direction Cosine Matrix ECEF to NED1/1 -> Invert 3x3 Matrix/1
  Direction Cosine Matrix ECI to ECEF/1 -> Invert 3x3 Matrix1/1
  Invert 3x3 Matrix/1 -> Matrix Multiply1/1  "NED to ECEF"
  Invert 3x3 Matrix1/1 -> Matrix Multiply2/1  "ECEF to ECI"
  Matrix Multiply1/1 -> Matrix Multiply2/2
  Matrix Multiply2/1 -> Quaternion Rotation/2  "ECI frame"
  q/1 -> Quaternion Rotation/1
  Quaternion Rotation/1 -> Matrix Multiply/2  "body frame"
  Multiply/1 -> Matrix Multiply1/2  "B_NED"

== system ReactionWheel/Reaction Wheels/T to w ==
  w_prev : Inport
  T : Inport  Port=2
  I : Inport  Port=3
  dT : Inport  Port=4
  Add : Sum
  Constant : Constant  Value=-1
  Divide : Product  Inputs=*/**
  w : Outport
  wires:
  T/1 -> Divide/1
  I/1 -> Divide/2
  dT/1 -> Divide/3
  Divide/1 -> Add/2
  w_prev/1 -> Add/1
  Add/1 -> w/1
  Constant/1 -> Divide/4

== system ReactionWheel/Reaction Wheels/deltaT ==
  Clock : Clock  Commented=on
  Constant : Constant  Commented=on  Value=0.01
  Constant1 : Constant
  Memory : Memory  Commented=on
  Min : MinMax  Commented=on  Function=max  Inputs=2
  Subtract : Sum  Commented=on  Inputs=+-
  dT : Outport
  wires:
  Clock/1 -> Memory/1, Subtract/1
  Memory/1 -> Subtract/2
  Subtract/1 -> Min/1
  Constant/1 -> Min/2
  Constant1/1 -> dT/1

== system ReactionWheel/Reaction Wheels/w to T ==
  w_f : Inport
  w_i : Inport  Port=2
  I : Inport  Port=3
  dT : Inport  Port=4
  Constant : Constant  Value=-1
  Divide : Product  Inputs=***/
  Subtract : Sum  Inputs=+-
  T : Outport
  wires:
  Constant/1 -> Divide/1
  I/1 -> Divide/2
  w_i/1 -> Subtract/2
  w_f/1 -> Subtract/1
  Subtract/1 -> Divide/3
  dT/1 -> Divide/4
  Divide/1 -> T/1

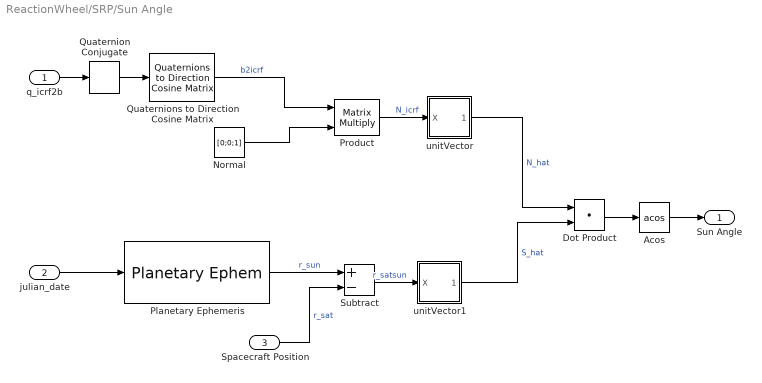
== system ReactionWheel/SRP/Sun Angle ==
  q_icrf2b : Inport
  julian_date : Inport  Port=2
  Spacecraft Position : Inport  Port=3
  Acos : Trigonometry  Operator=acos
  Dot Product : DotProduct  OutDataTypeStr=Inherit: Inherit via internal rule
  Normal : Constant  Value=[0;0;1]
  Planetary Ephemeris : PlanetaryEphem  units=m,m/s  ephemerisModel=DE432t  target=Sun  outputVelocity=off
  Product : Product  Multiplication=Matrix(*)
  Quaternion Conjugate : aerolibutil/Quaternion Conjugate
  Quaternions to Direction Cosine Matrix : sharedtransform/Quaternions to  Direction Cosine Matrix  aMode=aMode
      settings: LibrarySourceBlock=|
      | aerolibtransform2/Quaternions to
      | Direction Cosine Matrix
  Subtract : Sum  Inputs=+-
  unitVector : Subsystem
  unitVector1 : Subsystem
  Sun Angle : Outport
  wires:
  Normal/1 -> Product/2
  Quaternions to Direction Cosine Matrix/1 -> Product/1  "b2icrf"
  Spacecraft Position/1 -> Subtract/2  "r_sat"
  Planetary Ephemeris/1 -> Subtract/1  "r_sun"
  julian_date/1 -> Planetary Ephemeris/1
  Product/1 -> unitVector/1(X)  "N_icrf"
  Subtract/1 -> unitVector1/1(X)  "r_satsun"
  unitVector/1(X_hat) -> Dot Product/1  "N_hat"
  unitVector1/1(X_hat) -> Dot Product/2  "S_hat"
  Dot Product/1 -> Acos/1
  Acos/1 -> Sun Angle/1
  Quaternion Conjugate/1 -> Quaternions to Direction Cosine Matrix/1
  q_icrf2b/1 -> Quaternion Conjugate/1

== system ReactionWheel/icrf2lvlh/DCM_icrf2lvlh ==
  pos : Inport
  vel : Inport  Port=2
  Cross Product : matrix_library/Cross Product
  Cross Product1 : matrix_library/Cross Product
  Vector Concatenate : Concatenate  NumInputs=3  Mode=Multidimensional array  ConcatenateDimension=2
  unitVector : Subsystem
  unitVector1 : Subsystem
  unitVector2 : Subsystem
  DCM : Outport
  wires:
  pos/1 -> Cross Product/1, unitVector/1(X)
  unitVector/1(X_hat) -> Vector Concatenate/1, Cross Product1/2  "X_hat"
  vel/1 -> Cross Product/2
  Cross Product/1 -> unitVector1/1(X)  "h"
  unitVector1/1(X_hat) -> Vector Concatenate/3, Cross Product1/1  "Z_hat"
  Cross Product1/1 -> unitVector2/1(X)  "Y"
  unitVector2/1(X_hat) -> Vector Concatenate/2  "Y_hat"
  Vector Concatenate/1 -> DCM/1

== system ReactionWheel/Atmospheric Drag/Drag Angle/unitVector ==
  X : Inport
  Divide : Product  Inputs=*/
  Dot Product : DotProduct  OutDataTypeStr=Inherit: Inherit via internal rule
  Square Root : Sqrt
  X_hat : Outport
  wires:
  X/1 -> Divide/1, Dot Product/2, Dot Product/1
  Dot Product/1 -> Square Root/1
  Square Root/1 -> Divide/2
  Divide/1 -> X_hat/1

== system ReactionWheel/Atmospheric Drag/Drag Angle/unitVector1 ==
  X : Inport
  Divide : Product  Inputs=*/
  Dot Product : DotProduct  OutDataTypeStr=Inherit: Inherit via internal rule
  Square Root : Sqrt
  X_hat : Outport
  wires:
  X/1 -> Divide/1, Dot Product/2, Dot Product/1
  Dot Product/1 -> Square Root/1
  Square Root/1 -> Divide/2
  Divide/1 -> X_hat/1

== system ReactionWheel/CubeSat Animation/Antenna Position to VRML/ECEF to VRML ==
  M : Inport  PortDimensions=3
  Selector : Selector  InputPortWidth=3  IndexOptions=Index vector (dialog)  Indices=[2 3 1]  OutputSizes=1
  VR : Outport  PortDimensions=3  VectorParamsAs1DForOutWhenUnconnected=off
  wires:
  M/1 -> Selector/1
  Selector/1 -> VR/1

== system ReactionWheel/CubeSat Animation/Compute Earth Rotation Rate/Quaternion to VRML ==
  q : Inport
  Demux : Demux
  Gain : Gain  Gain=2
  Gain3 : Gain  Gain=[-1 1 1 1]
  Mux : Mux
  Selector : Selector  InputPortWidth=4  IndexOptions=Index vector (dialog)  Indices=[2 4 3 1]  OutputSizes=1
  Trigonometric Function : Trigonometry  Operator=acos
  AxisAngle : Outport  VectorParamsAs1DForOutWhenUnconnected=off
  wires:
  Demux/1 -> Trigonometric Function/1
  Trigonometric Function/1 -> Gain/1
  Mux/1 -> Selector/1
  q/1 -> Demux/1
  Gain3/1 -> AxisAngle/1
  Selector/1 -> Gain3/1
  Gain/1 -> Mux/1
  Demux/2 -> Mux/2
  Demux/3 -> Mux/3
  Demux/4 -> Mux/4

== system ReactionWheel/CubeSat Animation/Compute Umbra Translation/unitVec ==
  I : Inport
  Divide : Product  Inputs=*/
  Dot Product : DotProduct  OutDataTypeStr=Inherit: Inherit via internal rule
  Sqrt : Sqrt
  O : Outport  VectorParamsAs1DForOutWhenUnconnected=off
  wires:
  Dot Product/1 -> Sqrt/1
  I/1 -> Divide/1, Dot Product/1, Dot Product/2
  Divide/1 -> O/1
  Sqrt/1 -> Divide/2

== system ReactionWheel/CubeSat Animation/Sat Position to VRML/ECEF to VRML ==
  M : Inport  PortDimensions=3
  Selector : Selector  InputPortWidth=3  IndexOptions=Index vector (dialog)  Indices=[2 3 1]  OutputSizes=1
  VR : Outport  PortDimensions=3  VectorParamsAs1DForOutWhenUnconnected=off
  wires:
  M/1 -> Selector/1
  Selector/1 -> VR/1

== system ReactionWheel/CubeSat Animation/Sun Position to VRML/ECEF to VRML ==
  M : Inport  PortDimensions=3
  Selector : Selector  InputPortWidth=3  IndexOptions=Index vector (dialog)  Indices=[2 3 1]  OutputSizes=1
  VR : Outport  PortDimensions=3  VectorParamsAs1DForOutWhenUnconnected=off
  wires:
  M/1 -> Selector/1
  Selector/1 -> VR/1

== system ReactionWheel/Disturbance Torques/Atmospheric Drag Torque/Drag Angle ==
  q : Inport
  v : Inport  Port=2
  Acos : Trigonometry  Operator=acos
  Constant : Constant  Value=[0;0;1]
  Dot Product : DotProduct  OutDataTypeStr=Inherit: Inherit via internal rule
  Matrix Multiply : Product  Multiplication=Matrix(*)
  Quaternions to Direction Cosine Matrix : sharedtransform/Quaternions to  Direction Cosine Matrix  aMode=aMode
      settings: LibrarySourceBlock=|
      | aerolibtransform2/Quaternions to
      | Direction Cosine Matrix
  unitVector : Subsystem
  unitVector1 : Subsystem
  dragAngle : Outport
  wires:
  q/1 -> Quaternions to Direction Cosine Matrix/1
  Quaternions to Direction Cosine Matrix/1 -> Matrix Multiply/1
  v/1 -> Matrix Multiply/2
  Matrix Multiply/1 -> unitVector/1(X)  "v_body"
  Constant/1 -> unitVector1/1(X)
  unitVector/1(X_hat) -> Dot Product/1  "v_hat"
  unitVector1/1(X_hat) -> Dot Product/2  "N_hat"
  Dot Product/1 -> Acos/1
  Acos/1 -> dragAngle/1

== system ReactionWheel/SRP/Sun Angle/unitVector ==
  X : Inport
  Divide : Product  Inputs=*/
  Dot Product : DotProduct  OutDataTypeStr=Inherit: Inherit via internal rule
  Square Root : Sqrt
  X_hat : Outport
  wires:
  X/1 -> Divide/1, Dot Product/2, Dot Product/1
  Dot Product/1 -> Square Root/1
  Square Root/1 -> Divide/2
  Divide/1 -> X_hat/1

== system ReactionWheel/SRP/Sun Angle/unitVector1 ==
  X : Inport
  Divide : Product  Inputs=*/
  Dot Product : DotProduct  OutDataTypeStr=Inherit: Inherit via internal rule
  Square Root : Sqrt
  X_hat : Outport
  wires:
  X/1 -> Divide/1, Dot Product/2, Dot Product/1
  Dot Product/1 -> Square Root/1
  Square Root/1 -> Divide/2
  Divide/1 -> X_hat/1

== system ReactionWheel/icrf2lvlh/DCM_icrf2lvlh/unitVector ==
  X : Inport
  Divide : Product  Inputs=*/
  Dot Product : DotProduct  OutDataTypeStr=Inherit: Inherit via internal rule
  Square Root : Sqrt
  X_hat : Outport
  wires:
  X/1 -> Divide/1, Dot Product/2, Dot Product/1
  Dot Product/1 -> Square Root/1
  Square Root/1 -> Divide/2
  Divide/1 -> X_hat/1

== system ReactionWheel/icrf2lvlh/DCM_icrf2lvlh/unitVector1 ==
  X : Inport
  Divide : Product  Inputs=*/
  Dot Product : DotProduct  OutDataTypeStr=Inherit: Inherit via internal rule
  Square Root : Sqrt
  X_hat : Outport
  wires:
  X/1 -> Divide/1, Dot Product/2, Dot Product/1
  Dot Product/1 -> Square Root/1
  Square Root/1 -> Divide/2
  Divide/1 -> X_hat/1

== system ReactionWheel/icrf2lvlh/DCM_icrf2lvlh/unitVector2 ==
  X : Inport
  Divide : Product  Inputs=*/
  Dot Product : DotProduct  OutDataTypeStr=Inherit: Inherit via internal rule
  Square Root : Sqrt
  X_hat : Outport
  wires:
  X/1 -> Divide/1, Dot Product/2, Dot Product/1
  Dot Product/1 -> Square Root/1
  Square Root/1 -> Divide/2
  Divide/1 -> X_hat/1

== system ReactionWheel/Disturbance Torques/Atmospheric Drag Torque/Drag Angle/unitVector ==
  X : Inport
  Divide : Product  Inputs=*/
  Dot Product : DotProduct  OutDataTypeStr=Inherit: Inherit via internal rule
  Square Root : Sqrt
  X_hat : Outport
  wires:
  X/1 -> Divide/1, Dot Product/2, Dot Product/1
  Dot Product/1 -> Square Root/1
  Square Root/1 -> Divide/2
  Divide/1 -> X_hat/1

== system ReactionWheel/Disturbance Torques/Atmospheric Drag Torque/Drag Angle/unitVector1 ==
  X : Inport
  Divide : Product  Inputs=*/
  Dot Product : DotProduct  OutDataTypeStr=Inherit: Inherit via internal rule
  Square Root : Sqrt
  X_hat : Outport
  wires:
  X/1 -> Divide/1, Dot Product/2, Dot Product/1
  Dot Product/1 -> Square Root/1
  Square Root/1 -> Divide/2
  Divide/1 -> X_hat/1

== matlab function ReactionWheel/icrf2lvlh/MATLAB Function ==
  data: pos input; DCM output; vel input
function DCM = DCM_icrf2lvlh(pos,vel)

% Find unit vectors for creating DCM
X_hat = pos/vecnorm(pos); % direction of position vector
h = cross(pos,vel); 
Z_hat = h/vecnorm(h); % direction of + orbit normal
Y_hat = cross(Z_hat,X_hat); % direction of velocity 
Y_hat = Y_hat/vecnorm(Y_hat); % double check normalize

DCM = [X_hat, Y_hat, Z_hat];

% https://space.stackexchange.com/questions/33803/eci-to-lvlh-conversion
